simulink model "oloop3t"  (Simulink 2.09)
settings: Solver=ode45  StartTime=0.0  StopTime=120  MaxStep=1  RelTol=1e-7  AbsTol=1e-7
undefined symbols (not defined in the file or in its folder): Aac, Bac, Cac, Dac
settings Model: SaveTime=off  SaveOutput=off  ConsistencyChecking=off  RTWTemplateMakefile=grt_vc.tmf

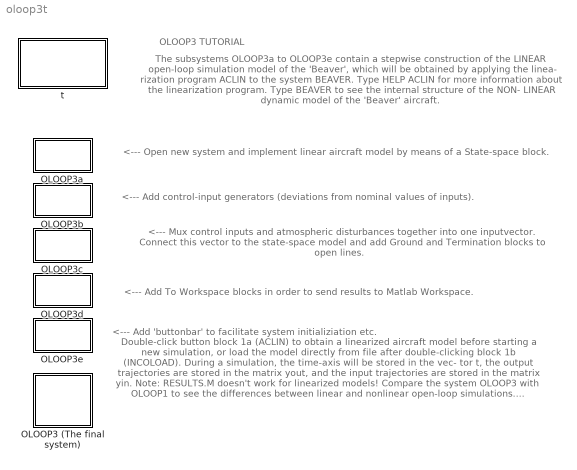
== system oloop3t ==
  note: <--- Mux control inputs and atmospheric disturbances together into one inputvector. Connect
      | this vector to the state-space model and add Ground and Termination blocks to open lines.
  note: <--- Add control-input generators (deviations from nominal values of inputs).
  note: OLOOP3 TUTORIAL
  note: The subsystems OLOOP3a to OLOOP3e contain a stepwise construction of the LINEAR
      | open-loop simulation model of the 'Beaver', which will be obtained by applying the linea-
      | rization program ACLIN to the system BEAVER. Type HELP ACLIN for more information
      | about the linearization program. Type BEAVER to see the internal structure of the NON-
      | LINEAR dynamic model of the 'Beaver' aircraft.
  note: <--- Open new system and implement linear aircraft model by means of a State-space block.
  note: <--- Add 'buttonbar' to facilitate system initializiation etc.
  note: <--- Add To Workspace blocks in order to send results to Matlab Workspace.
  note: Double-click button block 1a (ACLIN) to obtain a linearized aircraft model before
      | starting a new simulation, or load the model directly from file after double-clicking
      | block 1b (INCOLOAD). During a simulation, the time-axis will be stored in the vec-
      | tor t, the output trajectories are stored in the matrix yout, and the input trajectories
      | are stored in the matrix yin. Note: RESULTS.M doesn't work for linearized models!
      | Compare the system OLOOP3 with OLOOP1 to see the differences between linear
      | and nonlinear open-loop simulations. Remember that the linear model always uses
      | DEVIATIONS from nominal values of x, u, and y, whereas the nonlinear model
      | uses the real values (deviations + initial value).
  OLOOP3 (The final system) : Subsystem
      settings: OpenFcn=oloop3
  OLOOP3a : Subsystem
  OLOOP3b : Subsystem
  OLOOP3c : Subsystem
  OLOOP3d : Subsystem
  OLOOP3e : Subsystem
  t : Subsystem
      settings: OpenFcn=fdchelp oloop
      mask Display: disp('OLOOP3T\nMarc Rauw\nOctober 1997')

== system oloop3t/OLOOP3 (The final system) ==

== system oloop3t/OLOOP3a ==
  note: Step 2: take block State-space block from Simulink library 'linear'
  note: Step 3: specify Aac, Bac, Cac, and Dac to be state matrices of the linear model
      | (double-click the State-space block to do so)
  note: Step 1: open new system
  note: Construction of OLOOP3.
  Linear aircraft model : StateSpace  A=Aac  B=Bac  C=Cac  D=Dac  X0=0
  wires:
  ? -> Linear aircraft model/1
  Linear aircraft model/1 -> ?

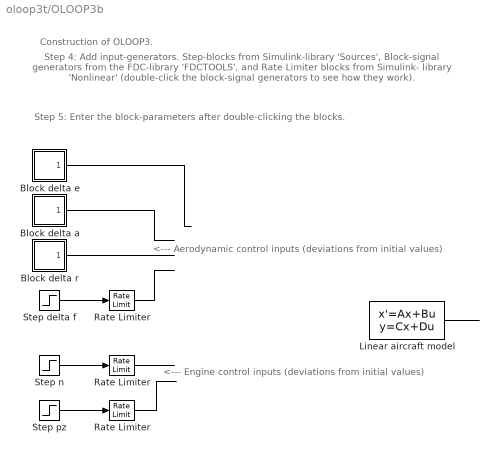
== system oloop3t/OLOOP3b ==
  note: <--- Engine control inputs
      | (deviations from initial values)
  note: <--- Aerodynamic control inputs
      | (deviations from initial values)
  note: Step 4: Add input-generators. Step-blocks from Simulink-library 'Sources', Block-signal
      | generators from the FDC-library 'FDCTOOLS', and Rate Limiter blocks from Simulink-
      | library 'Nonlinear' (double-click the block-signal generators to see how they work).
  note: Step 5: Enter the block-parameters after double-clicking the blocks.
  note: Construction of OLOOP3.
  " Rate Limiter" : RateLimiter  RisingSlewLimit=1.0  FallingSlewLimit=-1.0
  Block delta a : Subsystem  mask(Block Fcn){@1=0, @2=3*pi/180, @3=0, @4=2}
      mask prompts: @1 "Initial value (=final value):"; @2 "Amplitude of block (+ = step up, - = step down):"; @3 "Start time of block:"; @4 "Stop time of block:"
      mask help: Block Function
      mask init:
      | yinit=@1; yblock=@2; tstart=@3; tstop=@4;
      mask Help: This block implements a block signal.\nDefine the initial (=final) value, the\namplitude of the block (positive\n= upwards, negative=downwards),\nthe start time, and the stop time (must\nbe smaller than the start time).
      mask Display: plot(0,0,100,100,[100,60,60,20,20,0],[50,50,89,89,50,50])
  Block delta e : Subsystem  mask(Block Fcn){@1=0, @2=3*pi/180, @3=0, @4=2}
      mask prompts: @1 "Initial value (=final value):"; @2 "Amplitude of block (+ = step up, - = step down):"; @3 "Start time of block:"; @4 "Stop time of block:"
      mask help: Block Function
      mask init:
      | yinit=@1; yblock=@2; tstart=@3; tstop=@4;
      mask Help: This block implements a block signal.\nDefine the initial (=final) value, the\namplitude of the block (positive\n= upwards, negative=downwards),\nthe start time, and the stop time (must\nbe smaller than the start time).
      mask Display: plot(0,0,100,100,[100,60,60,20,20,0],[50,50,89,89,50,50])
  Block delta r : Subsystem  mask(Block Fcn){@1=0, @2=3*pi/180, @3=0, @4=2}
      mask prompts: @1 "Initial value (=final value):"; @2 "Amplitude of block (+ = step up, - = step down):"; @3 "Start time of block:"; @4 "Stop time of block:"
      mask help: Block Function
      mask init:
      | yinit=@1; yblock=@2; tstart=@3; tstop=@4;
      mask Help: This block implements a block signal.\nDefine the initial (=final) value, the\namplitude of the block (positive\n= upwards, negative=downwards),\nthe start time, and the stop time (must\nbe smaller than the start time).
      mask Display: plot(0,0,100,100,[100,60,60,20,20,0],[50,50,89,89,50,50])
  Linear aircraft model : StateSpace  A=Aac  B=Bac  C=Cac  D=Dac  X0=0
  Rate Limiter : RateLimiter  RisingSlewLimit=3*pi/180  FallingSlewLimit=-3*pi/180
  "Rate Limiter " : RateLimiter  RisingSlewLimit=50  FallingSlewLimit=-50
  Step delta f : Step  Time=0.001  Before=0  After=3*pi/180
  Step n : Step  Time=1  Before=0  After=200
  Step pz : Step  Time=0.001  Before=0  After=2
  wires:
  " Rate Limiter"/1 -> ?
  Rate Limiter/1 -> ?
  Block delta a/1(block) -> ?
  Block delta e/1(block) -> ?
  Step pz/1 -> " Rate Limiter"/1
  Step n/1 -> "Rate Limiter "/1
  Step delta f/1 -> Rate Limiter/1
  Block delta r/1(block) -> ?
  "Rate Limiter "/1 -> ?
  Linear aircraft model/1 -> ?
  ? -> Linear aircraft model/1

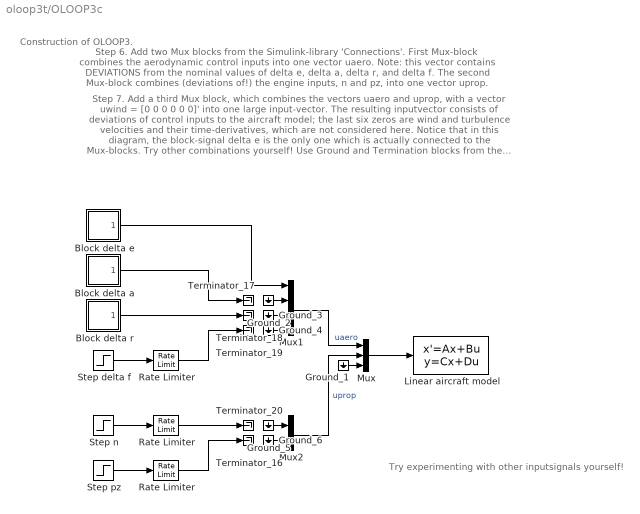
== system oloop3t/OLOOP3c ==
  note: Step 6. Add two Mux blocks from the Simulink-library 'Connections'. First Mux-block combines the aerodynamic control
      | inputs into one vector uaero. Note: this vector contains DEVIATIONS from the nominal values of delta e, delta a, delta r,
      | and delta f. The second Mux-block combines (deviations of!) the engine inputs, n and pz, into one vector uprop.
  note: Step 7. Add a third Mux block, which combines the vectors uaero and uprop, with a vector uwind = [0 0 0 0 0 0]' into one
      | large input-vector. The resulting inputvector consists of deviations of control inputs to the aircraft model; the last six zeros
      | are wind and turbulence velocities and their time-derivatives, which are not considered here. Notice that in this diagram,
      | the block-signal delta e is the only one which is actually connected to the Mux-blocks. Try other combinations yourself!
      | Use Ground and Termination blocks from the Simulink library Connections to end open lines (otherwise, Simulink will issue
      | warning messages during simulations).
  note: Try experimenting with other
      | inputsignals yourself!
  note: Construction of OLOOP3.
  " Rate Limiter" : RateLimiter  RisingSlewLimit=1.0  FallingSlewLimit=-1.0
  Block delta a : Subsystem  mask(Block Fcn){@1=0, @2=3*pi/180, @3=0, @4=2}
      mask prompts: @1 "Initial value (=final value):"; @2 "Amplitude of block (+ = step up, - = step down):"; @3 "Start time of block:"; @4 "Stop time of block:"
      mask help: Block Function
      mask init:
      | yinit=@1; yblock=@2; tstart=@3; tstop=@4;
      mask Help: This block implements a block signal.\nDefine the initial (=final) value, the\namplitude of the block (positive\n= upwards, negative=downwards),\nthe start time, and the stop time (must\nbe smaller than the start time).
      mask Display: plot(0,0,100,100,[100,60,60,20,20,0],[50,50,89,89,50,50])
  Block delta e : Subsystem  mask(Block Fcn){@1=0, @2=3*pi/180, @3=0, @4=2}
      mask prompts: @1 "Initial value (=final value):"; @2 "Amplitude of block (+ = step up, - = step down):"; @3 "Start time of block:"; @4 "Stop time of block:"
      mask help: Block Function
      mask init:
      | yinit=@1; yblock=@2; tstart=@3; tstop=@4;
      mask Help: This block implements a block signal.\nDefine the initial (=final) value, the\namplitude of the block (positive\n= upwards, negative=downwards),\nthe start time, and the stop time (must\nbe smaller than the start time).
      mask Display: plot(0,0,100,100,[100,60,60,20,20,0],[50,50,89,89,50,50])
  Block delta r : Subsystem  mask(Block Fcn){@1=0, @2=3*pi/180, @3=0, @4=2}
      mask prompts: @1 "Initial value (=final value):"; @2 "Amplitude of block (+ = step up, - = step down):"; @3 "Start time of block:"; @4 "Stop time of block:"
      mask help: Block Function
      mask init:
      | yinit=@1; yblock=@2; tstart=@3; tstop=@4;
      mask Help: This block implements a block signal.\nDefine the initial (=final) value, the\namplitude of the block (positive\n= upwards, negative=downwards),\nthe start time, and the stop time (must\nbe smaller than the start time).
      mask Display: plot(0,0,100,100,[100,60,60,20,20,0],[50,50,89,89,50,50])
  Ground_{1..6} (6 alike) : Ground
  Linear aircraft model : StateSpace  A=Aac  B=Bac  C=Cac  D=Dac  X0=0
  Mux : Mux  Inputs=[4 2 6]
  Mux1 : Mux  Inputs=4
  Mux2 : Mux  Inputs=2
  Rate Limiter : RateLimiter  RisingSlewLimit=3*pi/180  FallingSlewLimit=-3*pi/180
  "Rate Limiter " : RateLimiter  RisingSlewLimit=50  FallingSlewLimit=-50
  Step delta f : Step  Time=0.001  Before=0  After=3*pi/180
  Step n : Step  Time=1  Before=0  After=200
  Step pz : Step  Time=0.001  Before=0  After=2
  Terminator_{16..20} (5 alike) : Terminator
  wires:
  Mux/1 -> Linear aircraft model/1
  Mux1/1 -> Mux/1  "uaero"
  Mux2/1 -> Mux/2  "uprop"
  Ground_1/1 -> Mux/3
  " Rate Limiter"/1 -> Terminator_16/1
  "Rate Limiter "/1 -> Terminator_20/1
  Rate Limiter/1 -> Terminator_19/1
  Block delta r/1(block) -> Terminator_18/1
  Block delta a/1(block) -> Terminator_17/1
  Step delta f/1 -> Rate Limiter/1
  Step n/1 -> "Rate Limiter "/1
  Step pz/1 -> " Rate Limiter"/1
  Block delta e/1(block) -> Mux1/1
  Ground_2/1 -> Mux1/2
  Ground_3/1 -> Mux1/3
  Ground_4/1 -> Mux1/4
  Ground_5/1 -> Mux2/1
  Ground_6/1 -> Mux2/2

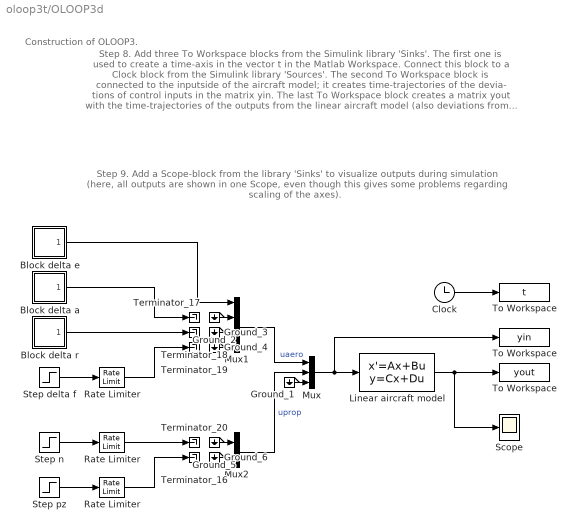
== system oloop3t/OLOOP3d ==
  note: Step 8. Add three To Workspace blocks from the Simulink library 'Sinks'. The first one is used to create a time-axis in
      | the vector t in the Matlab Workspace. Connect this block to a Clock block from the Simulink library 'Sources'. The
      | second To Workspace block is connected to the inputside of the aircraft model; it creates time-trajectories of the devia-
      | tions of control inputs in the matrix yin. The last To Workspace block creates a matrix yout with the time-trajectories of
      | the outputs from the linear aircraft model (also deviations from nominal values!). If the original system BEAVER is used
      | to obtain a linear state-space model, the outputvector will be: [ V alpha beta p q r psi theta phi xe ye H Hdot pb/2V ...
      | ... qc/V rb/2V]'  (see LEVEL1.HLP and the block-diagram of level1 of the system BEAVER).
  note: Step 9. Add a Scope-block from the library 'Sinks' to visualize outputs during simulation (here, all outputs are shown in
      | one Scope, even though this gives some problems regarding scaling of the axes).
  note: Construction of OLOOP3.
  " Rate Limiter" : RateLimiter  RisingSlewLimit=1.0  FallingSlewLimit=-1.0
  " To Workspace  " : ToWorkspace  VariableName=yin  SampleTime=0
      settings: Buffer=1000
  Block delta a : Subsystem  mask(Block Fcn){@1=0, @2=3*pi/180, @3=0, @4=2}
      mask prompts: @1 "Initial value (=final value):"; @2 "Amplitude of block (+ = step up, - = step down):"; @3 "Start time of block:"; @4 "Stop time of block:"
      mask help: Block Function
      mask init:
      | yinit=@1; yblock=@2; tstart=@3; tstop=@4;
      mask Help: This block implements a block signal.\nDefine the initial (=final) value, the\namplitude of the block (positive\n= upwards, negative=downwards),\nthe start time, and the stop time (must\nbe smaller than the start time).
      mask Display: plot(0,0,100,100,[100,60,60,20,20,0],[50,50,89,89,50,50])
  Block delta e : Subsystem  mask(Block Fcn){@1=0, @2=3*pi/180, @3=0, @4=2}
      mask prompts: @1 "Initial value (=final value):"; @2 "Amplitude of block (+ = step up, - = step down):"; @3 "Start time of block:"; @4 "Stop time of block:"
      mask help: Block Function
      mask init:
      | yinit=@1; yblock=@2; tstart=@3; tstop=@4;
      mask Help: This block implements a block signal.\nDefine the initial (=final) value, the\namplitude of the block (positive\n= upwards, negative=downwards),\nthe start time, and the stop time (must\nbe smaller than the start time).
      mask Display: plot(0,0,100,100,[100,60,60,20,20,0],[50,50,89,89,50,50])
  Block delta r : Subsystem  mask(Block Fcn){@1=0, @2=3*pi/180, @3=0, @4=2}
      mask prompts: @1 "Initial value (=final value):"; @2 "Amplitude of block (+ = step up, - = step down):"; @3 "Start time of block:"; @4 "Stop time of block:"
      mask help: Block Function
      mask init:
      | yinit=@1; yblock=@2; tstart=@3; tstop=@4;
      mask Help: This block implements a block signal.\nDefine the initial (=final) value, the\namplitude of the block (positive\n= upwards, negative=downwards),\nthe start time, and the stop time (must\nbe smaller than the start time).
      mask Display: plot(0,0,100,100,[100,60,60,20,20,0],[50,50,89,89,50,50])
  Clock : Clock
  Ground_{1..6} (6 alike) : Ground
  Linear aircraft model : StateSpace  A=Aac  B=Bac  C=Cac  D=Dac  X0=0
  Mux : Mux  Inputs=[4 2 6]
  Mux1 : Mux  Inputs=4
  Mux2 : Mux  Inputs=2
  Rate Limiter : RateLimiter  RisingSlewLimit=3*pi/180  FallingSlewLimit=-3*pi/180
  "Rate Limiter " : RateLimiter  RisingSlewLimit=50  FallingSlewLimit=-50
  Scope : Scope
      settings: TickLabels=on  TimeRange=120.000000  YMin=-50.000000  YMax=50.000000  SaveToWorkspace=off  SaveName=ScopeData
  Step delta f : Step  Time=0.001  Before=0  After=3*pi/180
  Step n : Step  Time=1  Before=0  After=200
  Step pz : Step  Time=0.001  Before=0  After=2
  Terminator_{16..20} (5 alike) : Terminator
  To Workspace : ToWorkspace  VariableName=t  SampleTime=0
      settings: Buffer=1000
  "To Workspace " : ToWorkspace  VariableName=yout  SampleTime=0
      settings: Buffer=1000
  wires:
  Ground_6/1 -> Mux2/2
  Ground_5/1 -> Mux2/1
  Ground_4/1 -> Mux1/4
  Ground_3/1 -> Mux1/3
  Ground_2/1 -> Mux1/2
  Block delta e/1(block) -> Mux1/1
  Step pz/1 -> " Rate Limiter"/1
  Step n/1 -> "Rate Limiter "/1
  Step delta f/1 -> Rate Limiter/1
  Clock/1 -> To Workspace/1
  Linear aircraft model/1 -> "To Workspace "/1, Scope/1
  Mux/1 -> Linear aircraft model/1, " To Workspace  "/1
  Block delta a/1(block) -> Terminator_17/1
  Block delta r/1(block) -> Terminator_18/1
  Rate Limiter/1 -> Terminator_19/1
  "Rate Limiter "/1 -> Terminator_20/1
  " Rate Limiter"/1 -> Terminator_16/1
  Ground_1/1 -> Mux/3
  Mux2/1 -> Mux/2  "uprop"
  Mux1/1 -> Mux/1  "uaero"

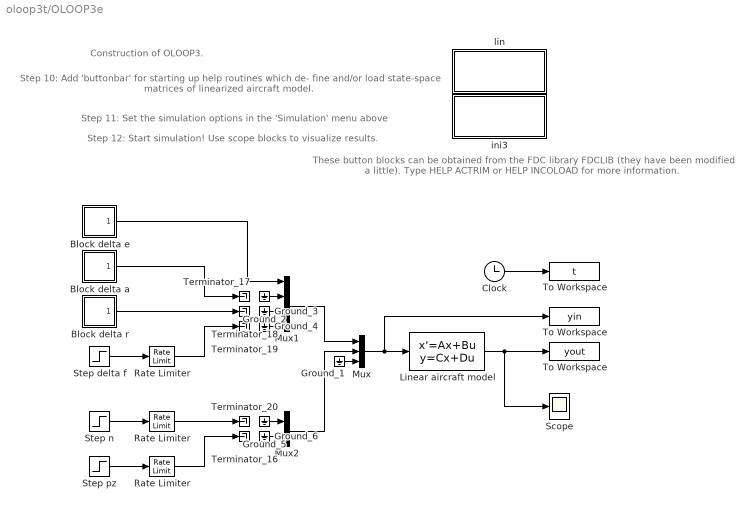
== system oloop3t/OLOOP3e ==
  note: Step 10: Add 'buttonbar' for starting up help routines which de-
      | fine and/or load state-space matrices of linearized aircraft model.
  note: Step 11: Set the simulation options in the 'Simulation' menu above
  note: Step 12: Start simulation! Use scope blocks to visualize results.
  note: These button  blocks can be obtained from
      | the FDC library FDCLIB (they have been
      | modified a little). Type HELP ACTRIM or
      | HELP INCOLOAD for more information.
  note: Construction of OLOOP3.
  " Rate Limiter" : RateLimiter  RisingSlewLimit=1.0  FallingSlewLimit=-1.0
  " To Workspace  " : ToWorkspace  VariableName=yin  SampleTime=0
      settings: Buffer=1000
  Block delta a : Subsystem  mask(Block Fcn){@1=0, @2=3*pi/180, @3=0, @4=2}
      mask prompts: @1 "Initial value (=final value):"; @2 "Amplitude of block (+ = step up, - = step down):"; @3 "Start time of block:"; @4 "Stop time of block:"
      mask help: Block Function
      mask init:
      | yinit=@1; yblock=@2; tstart=@3; tstop=@4;
      mask Help: This block implements a block signal.\nDefine the initial (=final) value, the\namplitude of the block (positive\n= upwards, negative=downwards),\nthe start time, and the stop time (must\nbe smaller than the start time).
      mask Display: plot(0,0,100,100,[100,60,60,20,20,0],[50,50,89,89,50,50])
  Block delta e : Subsystem  mask(Block Fcn){@1=0, @2=3*pi/180, @3=0, @4=2}
      mask prompts: @1 "Initial value (=final value):"; @2 "Amplitude of block (+ = step up, - = step down):"; @3 "Start time of block:"; @4 "Stop time of block:"
      mask help: Block Function
      mask init:
      | yinit=@1; yblock=@2; tstart=@3; tstop=@4;
      mask Help: This block implements a block signal.\nDefine the initial (=final) value, the\namplitude of the block (positive\n= upwards, negative=downwards),\nthe start time, and the stop time (must\nbe smaller than the start time).
      mask Display: plot(0,0,100,100,[100,60,60,20,20,0],[50,50,89,89,50,50])
  Block delta r : Subsystem  mask(Block Fcn){@1=0, @2=3*pi/180, @3=0, @4=2}
      mask prompts: @1 "Initial value (=final value):"; @2 "Amplitude of block (+ = step up, - = step down):"; @3 "Start time of block:"; @4 "Stop time of block:"
      mask help: Block Function
      mask init:
      | yinit=@1; yblock=@2; tstart=@3; tstop=@4;
      mask Help: This block implements a block signal.\nDefine the initial (=final) value, the\namplitude of the block (positive\n= upwards, negative=downwards),\nthe start time, and the stop time (must\nbe smaller than the start time).
      mask Display: plot(0,0,100,100,[100,60,60,20,20,0],[50,50,89,89,50,50])
  Clock : Clock
  Ground_{1..6} (6 alike) : Ground
  Linear aircraft model : StateSpace  A=Aac  B=Bac  C=Cac  D=Dac  X0=0
  Mux : Mux  Inputs=[4 2 6]
  Mux1 : Mux  Inputs=4
  Mux2 : Mux  Inputs=2
  Rate Limiter : RateLimiter  RisingSlewLimit=3*pi/180  FallingSlewLimit=-3*pi/180
  "Rate Limiter " : RateLimiter  RisingSlewLimit=50  FallingSlewLimit=-50
  Scope : Scope
      settings: TickLabels=on  TimeRange=120.000000  YMin=-50.000000  YMax=50.000000  SaveToWorkspace=off  SaveName=ScopeData
  Step delta f : Step  Time=0.001  Before=0  After=3*pi/180
  Step n : Step  Time=1  Before=0  After=200
  Step pz : Step  Time=0.001  Before=0  After=2
  Terminator_{16..20} (5 alike) : Terminator
  To Workspace : ToWorkspace  VariableName=t  SampleTime=0
      settings: Buffer=1000
  "To Workspace " : ToWorkspace  VariableName=yout  SampleTime=0
      settings: Buffer=1000
  ini3 : Subsystem
      settings: OpenFcn=incoload
      mask Type: incoload
      mask Display: disp('1b. Load linear\nmodel from file\nINCOLOAD')
  lin : Subsystem
      settings: OpenFcn=aclin
      mask Type: linearize aircraft model
      mask Display: disp('1a. Call lineari-\nzation routine\nACLIN')
  wires:
  Ground_6/1 -> Mux2/2
  Ground_5/1 -> Mux2/1
  Ground_4/1 -> Mux1/4
  Ground_3/1 -> Mux1/3
  Ground_2/1 -> Mux1/2
  Block delta e/1(block) -> Mux1/1
  Step pz/1 -> " Rate Limiter"/1
  Step n/1 -> "Rate Limiter "/1
  Step delta f/1 -> Rate Limiter/1
  Clock/1 -> To Workspace/1
  Linear aircraft model/1 -> "To Workspace "/1, Scope/1
  Mux/1 -> Linear aircraft model/1, " To Workspace  "/1
  Block delta a/1(block) -> Terminator_17/1
  Block delta r/1(block) -> Terminator_18/1
  Rate Limiter/1 -> Terminator_19/1
  "Rate Limiter "/1 -> Terminator_20/1
  " Rate Limiter"/1 -> Terminator_16/1
  Ground_1/1 -> Mux/3
  Mux2/1 -> Mux/2
  Mux1/1 -> Mux/1

== system oloop3t/t ==

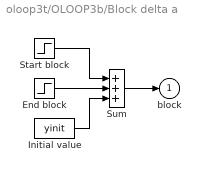
== system oloop3t/OLOOP3b/Block delta a ==
  End block : Step  Time=tstop  Before=0  After=-yblock
  Initial value : Constant  Value=yinit
  Start block : Step  Time=tstart  Before=0  After=yblock
  Sum : Sum  Inputs=+++
  block : Outport  Port=1  InitialOutput=0
  wires:
  End block/1 -> Sum/2
  Start block/1 -> Sum/1
  Initial value/1 -> Sum/3
  Sum/1 -> block/1

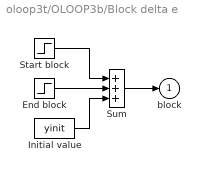
== system oloop3t/OLOOP3b/Block delta e ==
  End block : Step  Time=tstop  Before=0  After=-yblock
  Initial value : Constant  Value=yinit
  Start block : Step  Time=tstart  Before=0  After=yblock
  Sum : Sum  Inputs=+++
  block : Outport  Port=1  InitialOutput=0
  wires:
  Sum/1 -> block/1
  Initial value/1 -> Sum/3
  Start block/1 -> Sum/1
  End block/1 -> Sum/2

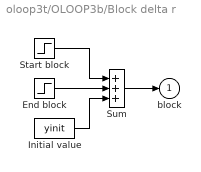
== system oloop3t/OLOOP3b/Block delta r ==
  End block : Step  Time=tstop  Before=0  After=-yblock
  Initial value : Constant  Value=yinit
  Start block : Step  Time=tstart  Before=0  After=yblock
  Sum : Sum  Inputs=+++
  block : Outport  Port=1  InitialOutput=0
  wires:
  Sum/1 -> block/1
  Initial value/1 -> Sum/3
  Start block/1 -> Sum/1
  End block/1 -> Sum/2

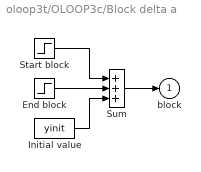
== system oloop3t/OLOOP3c/Block delta a ==
  End block : Step  Time=tstop  Before=0  After=-yblock
  Initial value : Constant  Value=yinit
  Start block : Step  Time=tstart  Before=0  After=yblock
  Sum : Sum  Inputs=+++
  block : Outport  Port=1  InitialOutput=0
  wires:
  Sum/1 -> block/1
  Initial value/1 -> Sum/3
  Start block/1 -> Sum/1
  End block/1 -> Sum/2

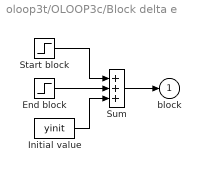
== system oloop3t/OLOOP3c/Block delta e ==
  End block : Step  Time=tstop  Before=0  After=-yblock
  Initial value : Constant  Value=yinit
  Start block : Step  Time=tstart  Before=0  After=yblock
  Sum : Sum  Inputs=+++
  block : Outport  Port=1  InitialOutput=0
  wires:
  End block/1 -> Sum/2
  Start block/1 -> Sum/1
  Initial value/1 -> Sum/3
  Sum/1 -> block/1

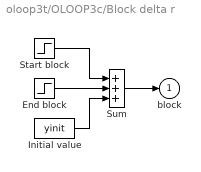
== system oloop3t/OLOOP3c/Block delta r ==
  End block : Step  Time=tstop  Before=0  After=-yblock
  Initial value : Constant  Value=yinit
  Start block : Step  Time=tstart  Before=0  After=yblock
  Sum : Sum  Inputs=+++
  block : Outport  Port=1  InitialOutput=0
  wires:
  End block/1 -> Sum/2
  Start block/1 -> Sum/1
  Initial value/1 -> Sum/3
  Sum/1 -> block/1

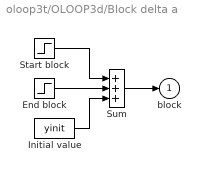
== system oloop3t/OLOOP3d/Block delta a ==
  End block : Step  Time=tstop  Before=0  After=-yblock
  Initial value : Constant  Value=yinit
  Start block : Step  Time=tstart  Before=0  After=yblock
  Sum : Sum  Inputs=+++
  block : Outport  Port=1  InitialOutput=0
  wires:
  End block/1 -> Sum/2
  Start block/1 -> Sum/1
  Initial value/1 -> Sum/3
  Sum/1 -> block/1

== system oloop3t/OLOOP3d/Block delta e ==
  End block : Step  Time=tstop  Before=0  After=-yblock
  Initial value : Constant  Value=yinit
  Start block : Step  Time=tstart  Before=0  After=yblock
  Sum : Sum  Inputs=+++
  block : Outport  Port=1  InitialOutput=0
  wires:
  Sum/1 -> block/1
  Initial value/1 -> Sum/3
  Start block/1 -> Sum/1
  End block/1 -> Sum/2

== system oloop3t/OLOOP3d/Block delta r ==
  End block : Step  Time=tstop  Before=0  After=-yblock
  Initial value : Constant  Value=yinit
  Start block : Step  Time=tstart  Before=0  After=yblock
  Sum : Sum  Inputs=+++
  block : Outport  Port=1  InitialOutput=0
  wires:
  Sum/1 -> block/1
  Initial value/1 -> Sum/3
  Start block/1 -> Sum/1
  End block/1 -> Sum/2

== system oloop3t/OLOOP3e/Block delta a ==
  End block : Step  Time=tstop  Before=0  After=-yblock
  Initial value : Constant  Value=yinit
  Start block : Step  Time=tstart  Before=0  After=yblock
  Sum : Sum  Inputs=+++
  block : Outport  Port=1  InitialOutput=0
  wires:
  End block/1 -> Sum/2
  Start block/1 -> Sum/1
  Initial value/1 -> Sum/3
  Sum/1 -> block/1

== system oloop3t/OLOOP3e/Block delta e ==
  End block : Step  Time=tstop  Before=0  After=-yblock
  Initial value : Constant  Value=yinit
  Start block : Step  Time=tstart  Before=0  After=yblock
  Sum : Sum  Inputs=+++
  block : Outport  Port=1  InitialOutput=0
  wires:
  Sum/1 -> block/1
  Initial value/1 -> Sum/3
  Start block/1 -> Sum/1
  End block/1 -> Sum/2

== system oloop3t/OLOOP3e/Block delta r ==
  End block : Step  Time=tstop  Before=0  After=-yblock
  Initial value : Constant  Value=yinit
  Start block : Step  Time=tstart  Before=0  After=yblock
  Sum : Sum  Inputs=+++
  block : Outport  Port=1  InitialOutput=0
  wires:
  Sum/1 -> block/1
  Initial value/1 -> Sum/3
  Start block/1 -> Sum/1
  End block/1 -> Sum/2

== system oloop3t/OLOOP3e/ini3 ==

== system oloop3t/OLOOP3e/lin ==
